simulink subsystem "ADC_To_Current"  (R2024b)
settings: Solver=VariableStepAuto  StartTime=0.0  StopTime=10.0  RelTol=1e-3
settings Model: Creator=JesseJabezArendse  LastModifiedBy=JesseJabezArendse

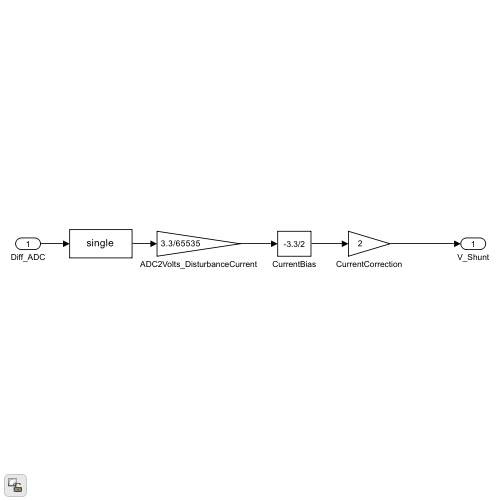
[thumbnail: Simulink's stored preview of the top-level diagram]
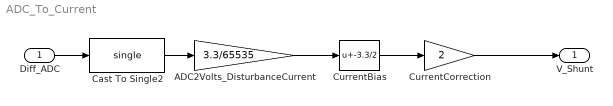
== system ADC_To_Current ==
  Diff_ADC : Inport  OutDataTypeStr=single
  ADC2Volts_DisturbanceCurrent : Gain  Gain=3.3/65535  OutDataTypeStr=single
  Cast To Single2 : DataTypeConversion  OutDataTypeStr=single  SaturateOnIntegerOverflow=off  RndMeth=Floor
  CurrentBias : Bias  Bias=-3.3/2  SaturateOnIntegerOverflow=off
  CurrentCorrection : Gain  Gain=2  OutDataTypeStr=single
  V_Shunt : Outport  OutDataTypeStr=single
  wires:
  Cast To Single2/1 -> ADC2Volts_DisturbanceCurrent/1
  Diff_ADC/1 -> Cast To Single2/1
  ADC2Volts_DisturbanceCurrent/1 -> CurrentBias/1
  CurrentCorrection/1 -> V_Shunt/1
  CurrentBias/1 -> CurrentCorrection/1
